simulink model "licenta_simulare"  (R2022a)
settings: Solver=VariableStepAuto  StartTime=0.0  StopTime=30  RelTol=1e-3
values from neighbouring files (symbols this model uses):
  A = [0 1 0 0 0 0 ... (first row only)    [licenta.m]    (also in licenta_G_T.m)
  Ae = [A E;0 0 0 0 0 0 0]    [licenta.m]
  B = [0 0 ... (first row only)    [licenta.m]    (also in licenta_G_T.m)
  Be = [B; 0 0]    [licenta.m]
  C = eye(6)    [licenta.m]    (also in licenta_G_T.m)
  Ce = [C [0;0;0;0;0;0]]    [licenta.m]
  E = [1;0;0;0;0;0]    [licenta.m]
  F = T*A-K1*C    [licenta.m]
  H = E*pinv(C*E)    [licenta.m]    (also in licenta_G_T.m = minreal(zpk(G*D)))
  K = place(A,B,poles*10)    [licenta.m]
  K_total = K1+K2    [licenta.m]
  L = place(A',C',poles)'    [licenta.m]
  L_extins = place(Ae',Ce',poles)'    [licenta.m]
settings Model: Creator=alexandra  LastModifiedBy=alexandra

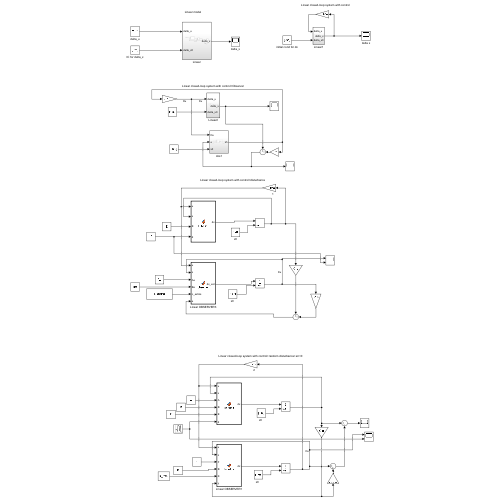
[thumbnail: Simulink's stored preview of the top-level diagram]
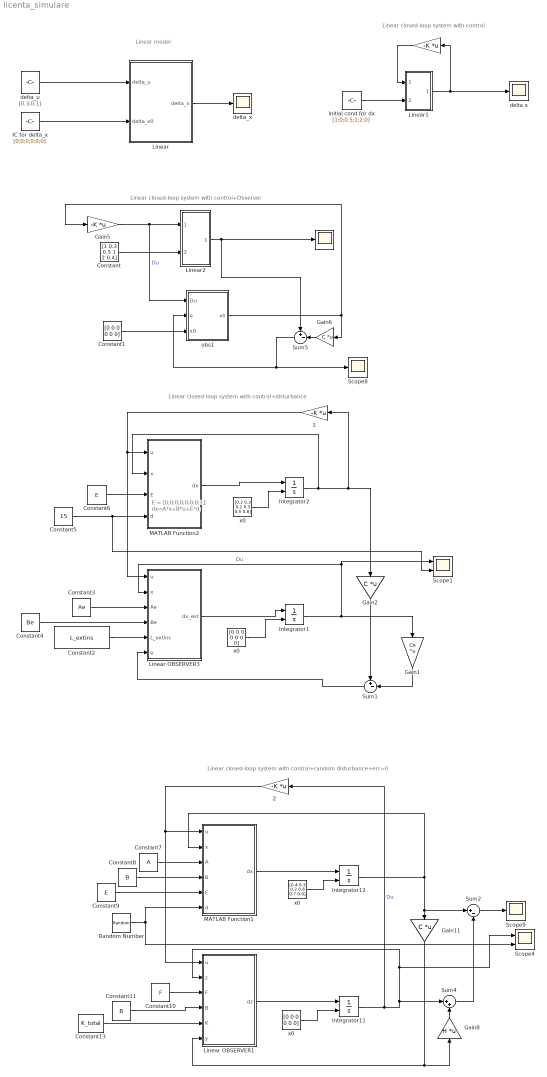
== system licenta_simulare ==
  note: E = [0;0;0;0;0;0;0;1];
      |
      | dx=A*x+B*u+E*d;
  note: Linear model
  note: Linear closed-loop system with control
  note: Linear closed-loop system with control+Observer
  note: Linear closed-loop system with control+disturbance
  note: Linear closed-loop system with control+random disturbance+err=0
  " " : Scope
  "         " : Gain  Gain=-K  Multiplication=Matrix(K*u)
  "         1" : Gain  Gain=-K  Multiplication=Matrix(K*u)
  "         2" : Gain  Gain=-K  Multiplication=Matrix(K*u)
  Constant : Constant  Value=[1 0.3 0.5 1 2 0.4]
  Constant1 : Constant  Value=[0 0 0 0 0 0]
  Constant10 : Constant  Value=F
  Constant11 : Constant  Value=B
  Constant13 : Constant  Value=K_total
  Constant2 : Constant  Value=L_extins
  Constant3 : Constant  Value=Ae
  Constant4 : Constant  Value=Be
  Constant5 : Constant  Value=15
  Constant6 : Constant  Value=E
  Constant7 : Constant  Value=A
  Constant8 : Constant  Value=B
  Constant9 : Constant  Value=E
  Gain1 : Gain  Gain=Ce  Multiplication=Matrix(K*u)
  Gain11 : Gain  Gain=C  Multiplication=Matrix(K*u)
  Gain2 : Gain  Gain=C  Multiplication=Matrix(K*u)
  Gain5 : Gain  Gain=-K  Multiplication=Matrix(K*u)
  Gain6 : Gain  Gain=C  Multiplication=Matrix(K*u)
  Gain8 : Gain  Gain=H  Multiplication=Matrix(K*u) (u vector)
  IC for delta_x : Constant  Value=[0;0;0;0;0;0]
  Integrator{1..2,11..12} (4 alike) : Integrator  InitialConditionSource=external  InitialCondition=[0 0 0 0]
  Linear : Subsystem
  Linear OBSERVER1 : MATLAB Function  TreatAsAtomicUnit=on
  Linear OBSERVER3 : MATLAB Function  TreatAsAtomicUnit=on
  Linear1 : Subsystem
  Linear2 : Subsystem
  MATLAB Function1 : MATLAB Function  TreatAsAtomicUnit=on
  MATLAB Function2 : MATLAB Function  TreatAsAtomicUnit=on
  Random Number : RandomNumber  Mean=2  SampleTime=0.1
  Scope1 : Scope  NumInputPorts=2
  Scope4 : Scope  NumInputPorts=2
  Scope8 : Scope
  Scope9 : Scope
  Sum1 : Sum  Inputs=+-|
  Sum2 : Sum  Inputs=|+-
  Sum4 : Sum  Inputs=|++
  Sum5 : Sum  Inputs=+-|
  "delta x " : Scope
  delta_u : Constant  Value=[0.3;0.1]
  delta_x : Scope
  initial cond for dx : Constant  Value=[1;0;0.5;1;2;0]
  obs1 : Subsystem
  x0 : Constant  Value=[0.2 0.3 0.2 0.3 0.5 0.8]
  "x0 " : Constant  Value=[0 0 0 0 0 0 0]
  "x0  " : Constant  Value=[0.4 0.3 0.2 0.6 0.7 0.9]
  "x0   " : Constant  Value=[0 0 0 0 0 0]
  wires:
  Linear1/1(delta_x) -> "delta x "/1, "         "/1
  initial cond for dx/1 -> Linear1/2(delta_x0)
  "         "/1 -> Linear1/1(delta_u)
  Linear/1(delta_x) -> delta_x/1
  IC for delta_x/1 -> Linear/2(delta_x0)
  delta_u/1 -> Linear/1(delta_u)
  Constant1/1 -> obs1/3(x0)
  obs1/1(xh) -> Gain5/1, Gain6/1
  Gain5/1 -> Linear2/1(delta_u), obs1/1(Du)  "Du"
  Constant/1 -> Linear2/2(delta_x0)
  Gain6/1 -> Sum5/2
  Linear2/1(delta_x) -> Sum5/1, " "/1
  Sum5/1 -> obs1/2(e), Scope8/1
  Gain2/1 -> Sum1/1
  Linear OBSERVER3/1(dx_est) -> Integrator1/1
  Sum1/1 -> Linear OBSERVER3/6(e)
  Constant5/1 -> Scope1/2, MATLAB Function2/4(d)
  x0/1 -> Integrator2/2
  MATLAB Function2/1(dx) -> Integrator2/1
  Integrator2/1 -> "         1"/1, Gain2/1, MATLAB Function2/2(x)
  Integrator1/1 -> Scope1/1, Linear OBSERVER3/2(x), Gain1/1  "Du"
  "x0 "/1 -> Integrator1/2
  "         1"/1 -> Linear OBSERVER3/1(u), MATLAB Function2/1(u)
  Gain1/1 -> Sum1/2
  Constant2/1 -> Linear OBSERVER3/5(L_extins)
  Constant3/1 -> Linear OBSERVER3/3(Ae)
  Constant4/1 -> Linear OBSERVER3/4(Be)
  Constant6/1 -> MATLAB Function2/3(E)
  Gain11/1 -> Linear OBSERVER1/6(y), Gain8/1
  Gain8/1 -> Sum4/2
  Linear OBSERVER1/1(dz) -> Integrator11/1
  "x0  "/1 -> Integrator12/2
  Sum4/1 -> Sum2/2
  Random Number/1 -> Scope4/2, MATLAB Function1/6(d)
  Integrator11/1 -> "         2"/1, Linear OBSERVER1/2(z), Scope4/1, Sum4/1  "Du"
  "x0   "/1 -> Integrator11/2
  "         2"/1 -> Linear OBSERVER1/1(u), MATLAB Function1/1(u)
  MATLAB Function1/1(dx) -> Integrator12/1
  Sum2/1 -> Scope9/1
  Integrator12/1 -> MATLAB Function1/2(x), Sum2/1, Gain11/1
  Constant9/1 -> MATLAB Function1/5(E)
  Constant8/1 -> MATLAB Function1/4(B)
  Constant7/1 -> MATLAB Function1/3(A)
  Constant10/1 -> Linear OBSERVER1/3(F)
  Constant11/1 -> Linear OBSERVER1/4(B)
  Constant13/1 -> Linear OBSERVER1/5(K)

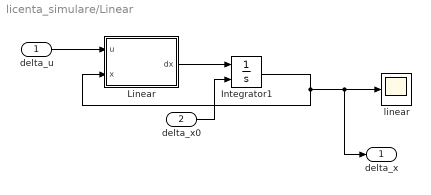
== system licenta_simulare/Linear ==
  delta_u : Inport
  delta_x0 : Inport  Port=2
  Integrator1 : Integrator  InitialConditionSource=external
  Linear : MATLAB Function  TreatAsAtomicUnit=on
  linear : Scope
  delta_x : Outport
  wires:
  Integrator1/1 -> Linear/2(x), delta_x/1, linear/1
  delta_u/1 -> Linear/1(u)
  Linear/1(dx) -> Integrator1/1
  delta_x0/1 -> Integrator1/2

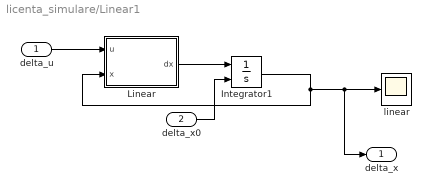
== system licenta_simulare/Linear1 ==
  delta_u : Inport
  delta_x0 : Inport  Port=2
  Integrator1 : Integrator  InitialConditionSource=external
  Linear : MATLAB Function  TreatAsAtomicUnit=on
  linear : Scope
  delta_x : Outport
  wires:
  Integrator1/1 -> Linear/2(x), delta_x/1, linear/1
  delta_u/1 -> Linear/1(u)
  Linear/1(dx) -> Integrator1/1
  delta_x0/1 -> Integrator1/2

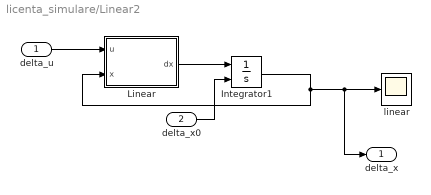
== system licenta_simulare/Linear2 ==
  delta_u : Inport
  delta_x0 : Inport  Port=2
  Integrator1 : Integrator  InitialConditionSource=external
  Linear : MATLAB Function  TreatAsAtomicUnit=on
  linear : Scope
  delta_x : Outport
  wires:
  Integrator1/1 -> Linear/2(x), delta_x/1, linear/1
  delta_u/1 -> Linear/1(u)
  Linear/1(dx) -> Integrator1/1
  delta_x0/1 -> Integrator1/2

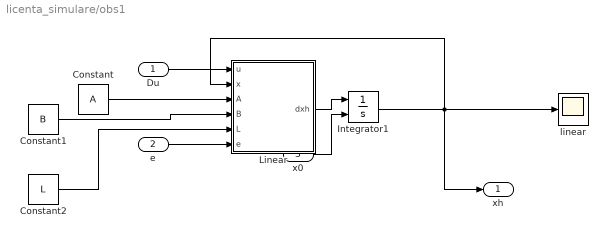
== system licenta_simulare/obs1 ==
  Du : Inport
  e : Inport  Port=2
  x0 : Inport  Port=3
  Constant : Constant  Value=A
  Constant1 : Constant  Value=B
  Constant2 : Constant  Value=L
  Integrator1 : Integrator  InitialConditionSource=external
  Linear : MATLAB Function  TreatAsAtomicUnit=on
  linear : Scope
  xh : Outport
  wires:
  Du/1 -> Linear/1(u)
  Linear/1(dxh) -> Integrator1/1
  x0/1 -> Integrator1/2
  Integrator1/1 -> xh/1, Linear/2(x), linear/1
  e/1 -> Linear/6(e)
  Constant/1 -> Linear/3(A)
  Constant1/1 -> Linear/4(B)
  Constant2/1 -> Linear/5(L)

== matlab function licenta_simulare/Linear1/Linear ==
  data: u input; dx output; x input
function dx = lin_fcn(u,x)

u1 = u(1);
u2 = u(2);

dx = [0;0;0;0;0;0];

dx(1)=x(2);
dx(2)=-0.4733*x(2)-29.1464*x(3)+0.4733*x(4)+109.3664*u1+109.3664*u2;
dx(3)=x(4);
dx(4)=0.1401*x(2)+29.1651*x(3)-0.1401*x(4)-32.3752*u1-32.3751*u2;
dx(5)=x(6);
dx(6)=-2.6349*x(6)-0.5055*u1+0.5055*u2;


dx = [dx(1) dx(2) dx(3) dx(4) dx(5) dx(6)]';

end

== matlab function licenta_simulare/Linear/Linear ==
  data: u input; dx output; x input
function dx = lin_fcn(u,x)

u1 = u(1);
u2 = u(2);

dx = [0;0;0;0;0;0];

dx(1)=x(2);
dx(2)=-0.4733*x(2)-29.1464*x(3)+0.4733*x(4)+109.3664*u1+109.3664*u2;
dx(3)=x(4);
dx(4)=0.1401*x(2)+29.1651*x(3)-0.1401*x(4)-32.3752*u1-32.3751*u2;
dx(5)=x(6);
dx(6)=-2.6349*x(6)-0.5055*u1+0.5055*u2;


dx = [dx(1) dx(2) dx(3) dx(4) dx(5) dx(6)]';

end

== matlab function licenta_simulare/Linear2/Linear ==
  data: u input; dx output; x input
function dx = lin_fcn(u,x)

u1 = u(1);
u2 = u(2);

dx = [0;0;0;0;0;0];

dx(1)=x(2);
dx(2)=-0.4733*x(2)-29.1464*x(3)+0.4733*x(4)+109.3664*u1+109.3664*u2;
dx(3)=x(4);
dx(4)=0.1401*x(2)+29.1651*x(3)-0.1401*x(4)-32.3752*u1-32.3751*u2;
dx(5)=x(6);
dx(6)=-2.6349*x(6)-0.5055*u1+0.5055*u2;


dx = [dx(1) dx(2) dx(3) dx(4) dx(5) dx(6)]';

end

== matlab function licenta_simulare/Linear OBSERVER3 ==
  data: u input; dx_est output; x input; Ae input; Be input; L_extins input; e input
function dx_est = observer(u,x,Ae,Be,L_extins,e)

 dx_est =Ae*x+Be*u+L_extins*e;

end

== matlab function licenta_simulare/MATLAB Function2 ==
  data: u input; dx output; x input; E input; d input
function dx   = liniarfcn(u,x,E,d)

A=[0 1 0 0 0 0;
    0 -0.4733 -29.1464 0.4733 0 0;
    0 0 0 1 0 0;
    0 0.1401 29.1651 -0.1401 0 0;
    0 0 0 0 0 1;
    0 0 0 0 0 -2.6349]
B=[0 0;
    109.3664 109.3664;
    0 0;
    -32.3752 -32.3752;
    0 0;
    -0.5055 0.5055]

dx=A*x+B*u+E*d;
end

== matlab function licenta_simulare/Linear OBSERVER1 ==
  data: u input; dz output; z input; F input; B input; K input; y input
function dz   = liniarfcn(u,z, F,B,K,y)
T=eye(6);
dz=F*z+T*B*u+K*y;
end

== matlab function licenta_simulare/MATLAB Function1 ==
  data: u input; dx output; x input; A input; B input; E input; d input
function dx   = liniarfcn(u,x,A,B,E,d)

dx=A*x+B*u+E*d;
end

== matlab function licenta_simulare/obs1/Linear ==
  data: u input; dxh output; x input; A input; B input; L input; e input
function dxh = obs_lin(u,x,A,B,L,e)

dxh = A*x + B*u + L*e;

end
